simulink model "plant_sovrastimato"  (R2020a)
settings: Solver=VariableStepAuto  StartTime=0.0  StopTime=10  MaxStep=1e-5  RelTol=1e-3
values from neighbouring files (symbols this model uses):
  Aa = 2    [dati_tesi_modellosimulink.m]
  g = 9.81    [dati_tesi_modellosimulink.m]
  l = 0.15    [dati_tesi_modellosimulink.m]
  L = 0.3    [dati_tesi_modellosimulink.m]
  lc = l/2    (= 0.075)    [dati_tesi_modellosimulink.m]
  Lc = L/2    (= 0.15)    [dati_tesi_modellosimulink.m]
  m = 2    [dati_tesi_modellosimulink.m]
  M = 4    [dati_tesi_modellosimulink.m]
  mc = 0    [dati_tesi_modellosimulink.m]
  Ra = 1    [dati_tesi_modellosimulink.m]
  wb = 2*pi*2    (= 12.5663706144)    [dati_tesi_modellosimulink.m]
libraries: fuzblock x7, simulink_extras x2, simulink x2
settings Model: Creator=Lucilla  LastModifiedBy=laura

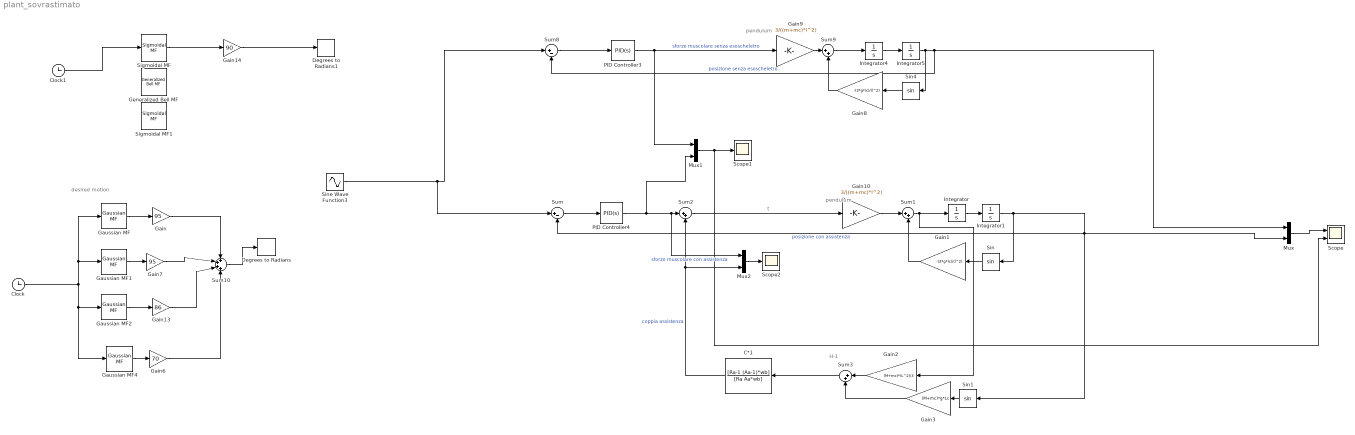
== system plant_sovrastimato ==
  note: desired motion
  note: H-1
  note: pendulum
  note: pendulum
  C*1 : TransferFcn  Numerator=[Ra-1 (Aa-1)*wb]  Denominator=[Ra Aa*wb]
  Clock : Clock
  Clock1 : Clock
  Degrees to Radians : simulink_extras/Transformations/Degrees to Radians
  Degrees to Radians1 : simulink_extras/Transformations/Degrees to Radians
  Gain : Gain  Gain=95
  Gain1 : Gain  Gain=-(3*g*lc)/(l^2)
  Gain10 : Gain  Gain=3/((m+mc)*l^2)
  Gain13 : Gain  Gain=86
  Gain14 : Gain  Gain=90
  Gain2 : Gain  Gain=(M+mc)*(L^2)/3
  Gain3 : Gain  Gain=(M+mc)*g*Lc
  Gain6 : Gain  Gain=70
  Gain7 : Gain  Gain=95
  Gain8 : Gain  Gain=-(3*g*lc)/(l^2)
  Gain9 : Gain  Gain=3/((m+mc)*l^2)
  Gaussian MF : fuzblock/Membership  Functions/Gaussian MF  sigma=0.4  mu=1.78
      settings: SourceProductBaseCode=FL
  Gaussian MF1 : fuzblock/Membership  Functions/Gaussian MF  sigma=0.4  mu=7
      settings: SourceProductBaseCode=FL
  Gaussian MF2 : fuzblock/Membership  Functions/Gaussian MF  sigma=0.38  mu=3.42
      settings: SourceProductBaseCode=FL
  Gaussian MF4 : fuzblock/Membership  Functions/Gaussian MF  sigma=0.32  mu=2.63
      settings: SourceProductBaseCode=FL
  Generalized Bell MF : fuzblock/Membership  Functions/Generalized Bell MF  a=1.5  b=4  c=6
      settings: SourceProductBaseCode=FL
  Integrator{,1,4..5} (4 alike) : Integrator
  Mux : Mux  Inputs=2
  Mux1 : Mux  Inputs=2
  Mux2 : Mux  Inputs=2
  PID Controller3 : simulink/Continuous/PID Controller  Controller=PID  Form=Parallel  TimeDomain=Continuous-time  UseExternalTs=off  SampleTime=-1  IntegratorMethod=Forward Euler  FilterMethod=Forward Euler  ControllerParametersSource=internal  P=20.396  I=105.7651  D=6.3413  UseFilter=on  N=150.7964  TunerSelectOption=Transfer Function Based (PID Tuner App)  InitialConditionSource=internal  InitialConditionForIntegrator=0  InitialConditionForFilter=0  DifferentiatorICPrevScaledInput=0  ExternalReset=none  TrackingMode=off  Kt=1  LimitOutput=off  UpperSaturationLimit=inf  LowerSaturationLimit=-inf  LinearizeAsGain=on  AntiWindupMode=none  Kb=1  POutMin=[]  POutMax=[]  IOutMin=[]  IOutMax=[]  DOutMin=[]  DOutMax=[]  NOutMin=[]  NOutMax=[]  SumOutMin=[]  SumOutMax=[]  SaturationOutMin=[]  SaturationOutMax=[]  PParamMin=[]  PParamMax=[]  IParamMin=[]  IParamMax=[]  DParamMin=[]  DParamMax=[]  NParamMin=[]  NParamMax=[]  KbParamMin=[]  KbParamMax=[]  KtParamMin=[]  KtParamMax=[]  KbOutMin=[]  KbOutMax=[]  KtOutMin=[]  KtOutMax=[]  IntegratorOutMin=[]  IntegratorOutMax=[]  FilterOutMin=[]  FilterOutMax=[]  SumI1OutMin=[]  SumI1OutMax=[]  SumI2OutMin=[]  SumI2OutMax=[]  SumI3OutMin=[]  SumI3OutMax=[]  SumI4OutMin=[]  SumI4OutMax=[]  SumDOutMin=[]  SumDOutMax=[]  DifferentiatorOutMin=[]  DifferentiatorOutMax=[]  FilterDiffOutCoefMin=[]  FilterDiffOutCoefMax=[]  ReciprocalOutMin=[]  ReciprocalOutMax=[]  SumDenOutMin=[]  SumDenOutMax=[]  SumNumOutMin=[]  SumNumOutMax=[]  DivideOutMin=[]  DivideOutMax=[]  UdiffTsProdOutMin=[]  UdiffTsProdOutMax=[]  NTsProdOutMin=[]  NTsProdOutMax=[]  UintegralTsProdOutMin=[]  UintegralTsProdOutMax=[]  UngainTsProdOutMin=[]  UngainTsProdOutMax=[]  IntegratorContinuousStateAttributes=''  IntegratorStateMustResolveToSignalObject=off  IntegratorRTWStateStorageClass=Auto  FilterContinuousStateAttributes=''  FilterStateMustResolveToSignalObject=off  FilterRTWStateStorageClass=Auto  ParallelPVariant=InternalParameters  IdealPVariant=Disabled  IVariant=InternalParameters  DVariant=InternalParameters  IntegratorVariant=Continuous  SatVariant=Disabled  AWVariant=Passthrough  PCopyVariant=Disabled  TRVariant=Disabled  FdbkBlocksVariant=Forward  IdealPFdbkVariant=Disabled  SatFdbkVariant=Disabled  DerivativeFilterVariant=ContFilter  NVariant=InternalParameters  NCopyVariant=Disabled  FilterICVariant=InternalICsFilter  IntegratorICVariant=InternalICs  ExternalResetVariant=Disabled  TRSumVariant=Passthrough  SumFdbkVariant=Disabled  SumVariant=Sum_PID  TsampFilterVariant=InternalTs  TsampNgainVariant=Passthrough  TsampIntegralVariant=Passthrough
  PID Controller4 : simulink/Continuous/PID Controller  Controller=PID  Form=Parallel  TimeDomain=Continuous-time  UseExternalTs=off  SampleTime=-1  IntegratorMethod=Forward Euler  FilterMethod=Forward Euler  ControllerParametersSource=internal  P=20.396  I=105.7651  D=6.3413  UseFilter=on  N=150.7964  TunerSelectOption=Transfer Function Based (PID Tuner App)  InitialConditionSource=internal  InitialConditionForIntegrator=0  InitialConditionForFilter=0  DifferentiatorICPrevScaledInput=0  ExternalReset=none  TrackingMode=off  Kt=1  LimitOutput=off  UpperSaturationLimit=inf  LowerSaturationLimit=-inf  LinearizeAsGain=on  AntiWindupMode=none  Kb=1  POutMin=[]  POutMax=[]  IOutMin=[]  IOutMax=[]  DOutMin=[]  DOutMax=[]  NOutMin=[]  NOutMax=[]  SumOutMin=[]  SumOutMax=[]  SaturationOutMin=[]  SaturationOutMax=[]  PParamMin=[]  PParamMax=[]  IParamMin=[]  IParamMax=[]  DParamMin=[]  DParamMax=[]  NParamMin=[]  NParamMax=[]  KbParamMin=[]  KbParamMax=[]  KtParamMin=[]  KtParamMax=[]  KbOutMin=[]  KbOutMax=[]  KtOutMin=[]  KtOutMax=[]  IntegratorOutMin=[]  IntegratorOutMax=[]  FilterOutMin=[]  FilterOutMax=[]  SumI1OutMin=[]  SumI1OutMax=[]  SumI2OutMin=[]  SumI2OutMax=[]  SumI3OutMin=[]  SumI3OutMax=[]  SumI4OutMin=[]  SumI4OutMax=[]  SumDOutMin=[]  SumDOutMax=[]  DifferentiatorOutMin=[]  DifferentiatorOutMax=[]  FilterDiffOutCoefMin=[]  FilterDiffOutCoefMax=[]  ReciprocalOutMin=[]  ReciprocalOutMax=[]  SumDenOutMin=[]  SumDenOutMax=[]  SumNumOutMin=[]  SumNumOutMax=[]  DivideOutMin=[]  DivideOutMax=[]  UdiffTsProdOutMin=[]  UdiffTsProdOutMax=[]  NTsProdOutMin=[]  NTsProdOutMax=[]  UintegralTsProdOutMin=[]  UintegralTsProdOutMax=[]  UngainTsProdOutMin=[]  UngainTsProdOutMax=[]  IntegratorContinuousStateAttributes=''  IntegratorStateMustResolveToSignalObject=off  IntegratorRTWStateStorageClass=Auto  FilterContinuousStateAttributes=''  FilterStateMustResolveToSignalObject=off  FilterRTWStateStorageClass=Auto  ParallelPVariant=InternalParameters  IdealPVariant=Disabled  IVariant=InternalParameters  DVariant=InternalParameters  IntegratorVariant=Continuous  SatVariant=Disabled  AWVariant=Passthrough  PCopyVariant=Disabled  TRVariant=Disabled  FdbkBlocksVariant=Forward  IdealPFdbkVariant=Disabled  SatFdbkVariant=Disabled  DerivativeFilterVariant=ContFilter  NVariant=InternalParameters  NCopyVariant=Disabled  FilterICVariant=InternalICsFilter  IntegratorICVariant=InternalICs  ExternalResetVariant=Disabled  TRSumVariant=Passthrough  SumFdbkVariant=Disabled  SumVariant=Sum_PID  TsampFilterVariant=InternalTs  TsampNgainVariant=Passthrough  TsampIntegralVariant=Passthrough
  Scope : Scope  NumInputPorts=2
  Scope1 : Scope
  Scope2 : Scope
  Sigmoidal MF : fuzblock/Membership  Functions/Sigmoidal MF  a=4  c=5
      settings: SourceProductBaseCode=FL
  Sigmoidal MF1 : fuzblock/Membership  Functions/Sigmoidal MF  a=-4  c=5
      settings: SourceProductBaseCode=FL
  Sin : Trigonometry
  Sin1 : Trigonometry
  Sin4 : Trigonometry
  Sine Wave Function3 : Sin  Frequency=55*pi*2  SampleTime=0
  Sum : Sum  Inputs=|+-
  Sum{1..3,9} (4 alike) : Sum  Inputs=|++
  Sum10 : Sum  Inputs=++++
  Sum8 : Sum  Inputs=|+-
  wires:
  Sum/1 -> PID Controller4/1
  Integrator1/1 -> Sin/1, Sin1/1, Mux/2, Sum/2  "posizione con assistenza"
  Gain10/1 -> Sum1/1
  Gain1/1 -> Sum1/2
  Sin/1 -> Gain1/1
  Integrator/1 -> Integrator1/1
  Sin1/1 -> Gain3/1
  Gain3/1 -> Sum3/2
  Gain2/1 -> Sum3/1
  Sum1/1 -> Integrator/1, Gain2/1
  PID Controller4/1 -> Mux1/2, Mux2/1, Sum2/1  "sforzo muscolare con assistenza"
  Sum2/1 -> Gain10/1  "t"
  Mux/1 -> Scope/1
  Mux1/1 -> Scope/2, Scope1/1
  Sum9/1 -> Integrator4/1
  Integrator4/1 -> Integrator5/1
  Sin4/1 -> Gain8/1
  Gain8/1 -> Sum9/2
  Gain9/1 -> Sum9/1
  Integrator5/1 -> Mux/1, Sum8/2, Sin4/1  "posizione senza esoscheletro"
  Gain6/1 -> Sum10/4
  Gaussian MF4/1 -> Gain6/1
  Gaussian MF/1 -> Gain/1
  Clock/1 -> Gaussian MF/1, Gaussian MF1/1, Gaussian MF4/1, Gaussian MF2/1
  Gain/1 -> Sum10/1
  Gaussian MF1/1 -> Gain7/1
  Gain7/1 -> Sum10/2
  Gaussian MF2/1 -> Gain13/1
  Gain13/1 -> Sum10/3
  Sum10/1 -> Degrees to Radians/1
  PID Controller3/1 -> Mux1/1, Gain9/1  "sforzo muscolare senza esoscheletro"
  Sum8/1 -> PID Controller3/1
  Gain14/1 -> Degrees to Radians1/1
  Sum3/1 -> C*1/1
  C*1/1 -> Mux2/2, Sum2/2  "coppia assistenza"
  Sigmoidal MF/1 -> Gain14/1
  Clock1/1 -> Sigmoidal MF/1
  Mux2/1 -> Scope2/1
  Sine Wave Function3/1 -> Sum/1, Sum8/1
